simulink model "host_firmware_NVH_v6"  (R2022a)
settings: Solver=VariableStepAuto  StartTime=0.0  StopTime=Inf  RelTol=1e-3
InitFcn:
  | params_NVH;
undefined symbols (not defined in the file): denz, numz, Ts
libraries: simulink x8, instrumentseriallib x3
settings Model: Creator=Renato  LastModifiedBy=Renato
settings SolverCC: AlgebraicLoopSolver=TrustRegion
settings DebuggingCC: UnconnectedInputMsg=warning  UnconnectedOutputMsg=warning  UnconnectedLineMsg=warning  SFMachineParentedDataDiag=warning
settings RTWCC: DLArmComputeVersion=19.05

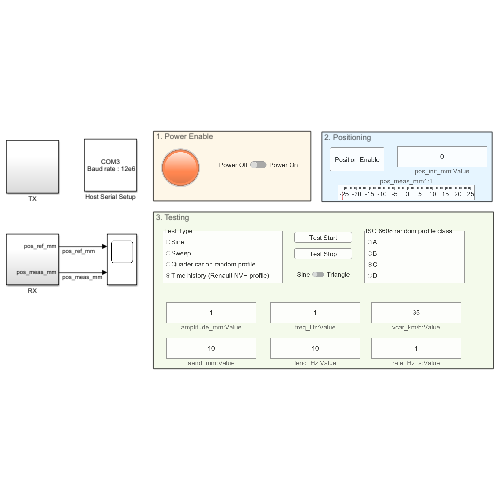
[thumbnail: Simulink's stored preview of the top-level diagram]
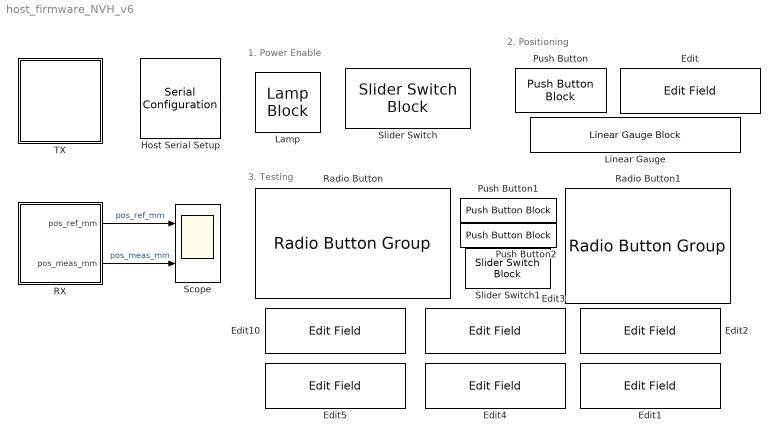
== system host_firmware_NVH_v6 ==
  note: 3. Testing
  note: 1. Power Enable
  note: 2. Positioning
  Edit{,1..5,10} (7 alike) : EditField  LabelPosition=Bottom  ShowInitialText=on  Alignment=Center
  Host Serial Setup : instrumentseriallib/Serial Configuration  Priority=-99  PortSel=COM3  Port=COM3  ComPort=COM3  BaudRate=12e6  DataBits=8  Parity=none  StopBits=1  ByteOrder=little-endian  FlowControl=none  Timeout=2  SimulateUsing=Interpreted execution  BlockInModel=on  aMode=5
      settings: SourceProductBaseCode=OT,IC,MT
  Lamp : LampBlock  LabelPosition=Hide
  Linear Gauge : LinearGaugeBlock  ScaleMin=-25  ScaleMax=25  TickInterval=5
  Push Button : PushButtonBlock  ButtonText=Position Enable  OffValue=0.000000
  Push Button1 : PushButtonBlock  ButtonText=Test Start  OffValue=0.000000
  Push Button2 : PushButtonBlock  ButtonText=Test Stop  OffValue=0.000000
  RX : Subsystem
  Radio Button : RadioButtonGroup  LabelPosition=Hide  SelectedLabel=Time history (Renault NVH profile)  ButtonGroupName=Test Type
      settings: Values={{'Sine', 'Sweep', 'Quarter car on random profile', 'Time history (Renault NVH profile)'}, [0 1 2 3]}
  Radio Button1 : RadioButtonGroup  LabelPosition=Hide  SelectedLabel=C  ButtonGroupName=ISO 8608 random profile class
      settings: Values={{'A', 'B', 'C', 'D'}, [0 1 2 3]}
  Scope : Scope  NumInputPorts=2
  Slider Switch : SliderSwitchBlock  LabelPosition=Hide
      settings: Values={{'Power Off', 'Power On'}, [0 1]}
  Slider Switch1 : SliderSwitchBlock  LabelPosition=Hide
      settings: Values={{'Sine', 'Triangle'}, [0 1]}
  TX : Subsystem
  wires:
  RX/1(pos_ref_mm) -> Scope/1  "pos_ref_mm"
  RX/2(pos_meas_mm) -> Scope/2  "pos_meas_mm"

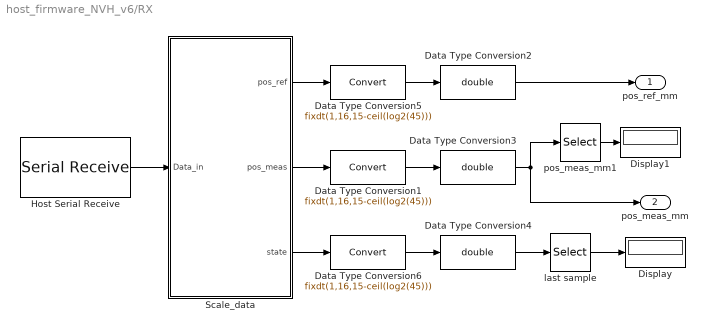
== system host_firmware_NVH_v6/RX ==
  Data Type Conversion1 : DataTypeConversion  OutDataTypeStr=fixdt(1,16,15-ceil(log2(45)))  ConvertRealWorld=Stored Integer (SI)  RndMeth=Simplest  SaturateOnIntegerOverflow=off
  Data Type Conversion2 : DataTypeConversion  OutDataTypeStr=double  RndMeth=Simplest  SaturateOnIntegerOverflow=off
  Data Type Conversion3 : DataTypeConversion  OutDataTypeStr=double  RndMeth=Simplest  SaturateOnIntegerOverflow=off
  Data Type Conversion4 : DataTypeConversion  OutDataTypeStr=double  RndMeth=Simplest  SaturateOnIntegerOverflow=off
  Data Type Conversion5 : DataTypeConversion  OutDataTypeStr=fixdt(1,16,15-ceil(log2(45)))  ConvertRealWorld=Stored Integer (SI)  RndMeth=Simplest  SaturateOnIntegerOverflow=off
  Data Type Conversion6 : DataTypeConversion  OutDataTypeStr=fixdt(1,16,15-ceil(log2(45)))  ConvertRealWorld=Stored Integer (SI)  RndMeth=Simplest  SaturateOnIntegerOverflow=off
  Display : Display
  Display1 : Display
  Host Serial Receive : instrumentseriallib/Serial Receive  PortSel=COM3  Port=COM3  ComPort=COM3  DataType=uint16  SaveDataType=uint8  ToggleHeader=on  Header='SS'  ToggleTerminator=on  Terminator=Custom terminator  CustomTerminator='EE'  InputFormat=Row major  ToggleDataSize=on  DataSize=[1000 3]  EnableBlockingMode=on  ActionDataUnavailable=Output last received value  ActionWhenDataUnavailable=Output last received value  CustomValue=0  SampleTime=1000 * Ts  SimulateUsing=Interpreted execution  BlockInModel=on  aMode=5
      settings: SourceProductBaseCode=OT,IC,MT
  Scale_data : MATLAB Function  TreatAsAtomicUnit=on
  last sample : Selector  NumberOfDimensions=2  InputPortWidth=3  IndexOptions=Index vector (dialog),Starting index (dialog)  Indices=1000,1  OutputSizes=1,1
  pos_meas_mm1 : Selector  NumberOfDimensions=2  InputPortWidth=3  IndexOptions=Index vector (dialog),Starting index (dialog)  Indices=1000,1  OutputSizes=1,1
  pos_ref_mm : Outport
  pos_meas_mm : Outport  Port=2
  wires:
  Host Serial Receive/1 -> Scale_data/1(Data_in)
  Scale_data/3(state) -> Data Type Conversion6/1
  Scale_data/2(pos_meas) -> Data Type Conversion1/1
  Scale_data/1(pos_ref) -> Data Type Conversion5/1
  Data Type Conversion5/1 -> Data Type Conversion2/1
  Data Type Conversion1/1 -> Data Type Conversion3/1
  Data Type Conversion2/1 -> pos_ref_mm/1
  Data Type Conversion3/1 -> pos_meas_mm1/1, pos_meas_mm/1
  Data Type Conversion4/1 -> last sample/1
  Data Type Conversion6/1 -> Data Type Conversion4/1
  last sample/1 -> Display/1
  pos_meas_mm1/1 -> Display1/1

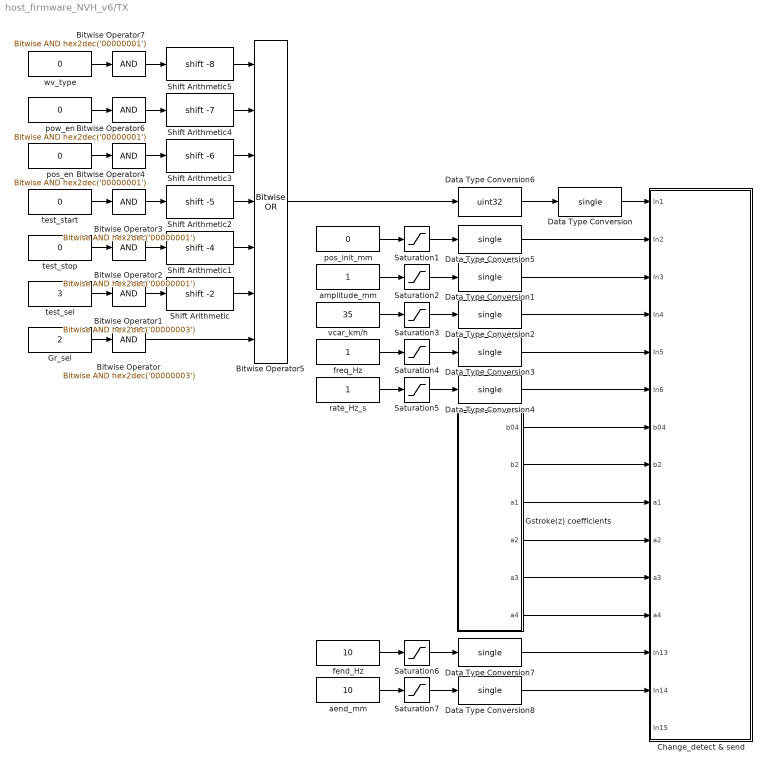
== system host_firmware_NVH_v6/TX ==
  Bitwise Operator : simulink/Logic and Bit Operations/Bitwise Operator  logicop=AND  UseBitMask=on  BitMask=hex2dec('00000003')  BitMaskRealWorld=Stored Integer
  Bitwise Operator1 : simulink/Logic and Bit Operations/Bitwise Operator  logicop=AND  UseBitMask=on  BitMask=hex2dec('00000003')  BitMaskRealWorld=Stored Integer
  Bitwise Operator{2..4,6..7} (5 alike) : simulink/Logic and Bit Operations/Bitwise Operator  logicop=AND  UseBitMask=on  BitMask=hex2dec('00000001')  BitMaskRealWorld=Stored Integer
  Bitwise Operator5 : simulink/Logic and Bit Operations/Bitwise Operator  logicop=OR  UseBitMask=off  NumInputPorts=7  BitMask=bin2dec('11011001')  BitMaskRealWorld=Stored Integer
  Change_detect & send : Subsystem
  Data Type Conversion : DataTypeConversion  OutDataTypeStr=single  ConvertRealWorld=Stored Integer (SI)  SaturateOnIntegerOverflow=off  RndMeth=Floor
  Data Type Conversion{1..5,7..8} (7 alike) : DataTypeConversion  OutDataTypeStr=single  RndMeth=Simplest  SaturateOnIntegerOverflow=off
  Data Type Conversion6 : DataTypeConversion  OutDataTypeStr=uint32  RndMeth=Simplest  SaturateOnIntegerOverflow=off
  Gr_sel : Constant  Value=2  VectorParams1D=off  OutDataTypeStr=uint32  SampleTime=0.01
  Gstroke(z) coefficients : Subsystem
  Saturation1 : Saturate  UpperLimit=20  LowerLimit=-20
  Saturation2 : Saturate  UpperLimit=20  LowerLimit=0
  Saturation3 : Saturate  UpperLimit=200  LowerLimit=10
  Saturation4 : Saturate  UpperLimit=100  LowerLimit=0.1
  Saturation5 : Saturate  UpperLimit=10  LowerLimit=0.1
  Saturation6 : Saturate  UpperLimit=100  LowerLimit=0.1
  Saturation7 : Saturate  UpperLimit=20  LowerLimit=0
  Shift Arithmetic : ArithShift  BitShiftNumber=-2
  Shift Arithmetic1 : ArithShift  BitShiftNumber=-4
  Shift Arithmetic2 : ArithShift  BitShiftNumber=-5
  Shift Arithmetic3 : ArithShift  BitShiftNumber=-6
  Shift Arithmetic4 : ArithShift  BitShiftNumber=-7
  Shift Arithmetic5 : ArithShift  BitShiftNumber=-8
  aend_mm : Constant  Value=10  VectorParams1D=off  OutDataTypeStr=single  SampleTime=0.01
  amplitude_mm : Constant  VectorParams1D=off  OutDataTypeStr=single  SampleTime=0.01
  fend_Hz : Constant  Value=10  VectorParams1D=off  OutDataTypeStr=single  SampleTime=0.01
  freq_Hz : Constant  VectorParams1D=off  OutDataTypeStr=single  SampleTime=0.01
  pos_en : Constant  Value=0  VectorParams1D=off  OutDataTypeStr=uint32  SampleTime=0.01
  pos_init_mm : Constant  Value=0  VectorParams1D=off  OutDataTypeStr=single  SampleTime=0.01
  pow_en : Constant  Value=0  VectorParams1D=off  OutDataTypeStr=uint32  SampleTime=0.01
  rate_Hz_s : Constant  VectorParams1D=off  OutDataTypeStr=single  SampleTime=0.01
  test_sel : Constant  Value=3  VectorParams1D=off  OutDataTypeStr=uint32  SampleTime=0.01
  test_start : Constant  Value=0  VectorParams1D=off  OutDataTypeStr=uint32  SampleTime=0.01
  test_stop : Constant  Value=0  VectorParams1D=off  OutDataTypeStr=uint32  SampleTime=0.01
  vcar_km/h : Constant  Value=35  VectorParams1D=off  OutDataTypeStr=single  SampleTime=0.01
  wv_type : Constant  Value=0  VectorParams1D=off  OutDataTypeStr=uint32  SampleTime=0.01
  wires:
  test_sel/1 -> Bitwise Operator1/1
  Gr_sel/1 -> Bitwise Operator/1
  Bitwise Operator1/1 -> Shift Arithmetic/1
  test_stop/1 -> Bitwise Operator2/1
  test_start/1 -> Bitwise Operator3/1
  pos_en/1 -> Bitwise Operator4/1
  pow_en/1 -> Bitwise Operator6/1
  Bitwise Operator2/1 -> Shift Arithmetic1/1
  Bitwise Operator3/1 -> Shift Arithmetic2/1
  Bitwise Operator4/1 -> Shift Arithmetic3/1
  Bitwise Operator6/1 -> Shift Arithmetic4/1
  pos_init_mm/1 -> Saturation1/1
  amplitude_mm/1 -> Saturation2/1
  vcar_km/h/1 -> Saturation3/1
  freq_Hz/1 -> Saturation4/1
  Saturation2/1 -> Data Type Conversion1/1
  Saturation3/1 -> Data Type Conversion2/1
  Saturation4/1 -> Data Type Conversion3/1
  Saturation1/1 -> Data Type Conversion5/1
  Bitwise Operator5/1 -> Data Type Conversion6/1
  Data Type Conversion/1 -> Change_detect & send/1(In1)
  Saturation5/1 -> Data Type Conversion4/1
  rate_Hz_s/1 -> Saturation5/1
  Data Type Conversion5/1 -> Change_detect & send/2(In2)
  Data Type Conversion1/1 -> Change_detect & send/3(In3)
  Data Type Conversion2/1 -> Change_detect & send/4(In4)
  Data Type Conversion3/1 -> Change_detect & send/5(In5)
  Data Type Conversion4/1 -> Change_detect & send/6(In6)
  Gstroke(z) coefficients/1(b04) -> Change_detect & send/7(b04)
  Gstroke(z) coefficients/2(b2) -> Change_detect & send/8(b2)
  Gstroke(z) coefficients/3(a1) -> Change_detect & send/9(a1)
  Gstroke(z) coefficients/4(a2) -> Change_detect & send/10(a2)
  Gstroke(z) coefficients/5(a3) -> Change_detect & send/11(a3)
  Gstroke(z) coefficients/6(a4) -> Change_detect & send/12(a4)
  Data Type Conversion6/1 -> Data Type Conversion/1
  Data Type Conversion7/1 -> Change_detect & send/13(In13)
  Saturation6/1 -> Data Type Conversion7/1
  fend_Hz/1 -> Saturation6/1
  Data Type Conversion8/1 -> Change_detect & send/14(In14)
  aend_mm/1 -> Saturation7/1
  Saturation7/1 -> Data Type Conversion8/1
  Bitwise Operator/1 -> Bitwise Operator5/7
  wv_type/1 -> Bitwise Operator7/1
  Bitwise Operator7/1 -> Shift Arithmetic5/1
  Shift Arithmetic5/1 -> Bitwise Operator5/1
  Shift Arithmetic4/1 -> Bitwise Operator5/2
  Shift Arithmetic3/1 -> Bitwise Operator5/3
  Shift Arithmetic2/1 -> Bitwise Operator5/4
  Shift Arithmetic1/1 -> Bitwise Operator5/5
  Shift Arithmetic/1 -> Bitwise Operator5/6

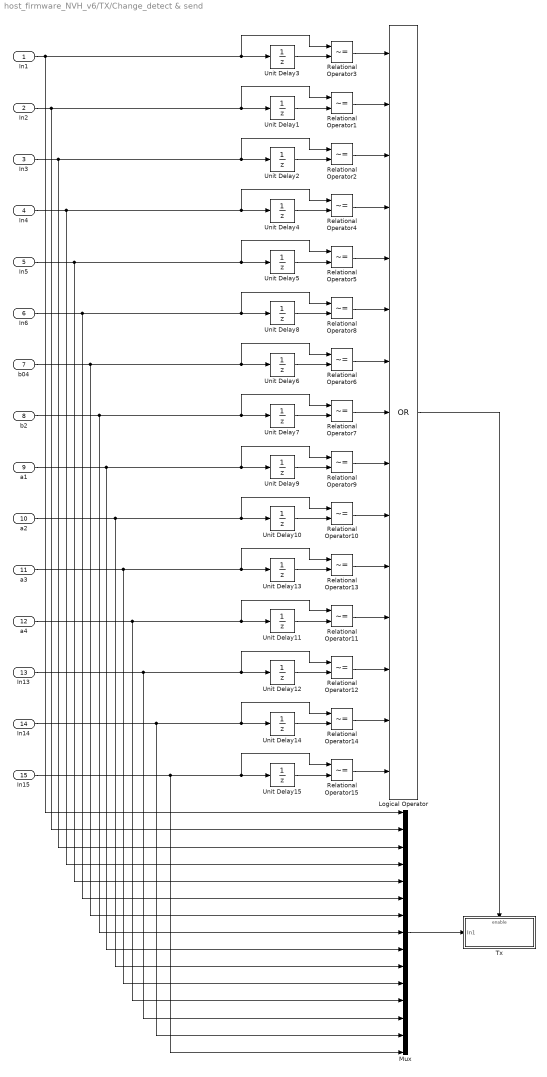
== system host_firmware_NVH_v6/TX/Change_detect & send ==
  In1 : Inport
  In2 : Inport  Port=2
  In3 : Inport  Port=3
  In4 : Inport  Port=4
  In5 : Inport  Port=5
  In6 : Inport  Port=6
  b04 : Inport  Port=7
  b2 : Inport  Port=8
  a1 : Inport  Port=9
  a2 : Inport  Port=10
  a3 : Inport  Port=11
  a4 : Inport  Port=12
  In13 : Inport  Port=13
  In14 : Inport  Port=14
  In15 : Inport  Port=15
  Logical Operator : Logic  Operator=OR  Inputs=15  AllPortsSameDT=off  OutDataTypeStr=boolean
  Mux : Mux  Inputs=15
  Relational Operator{1..15} (15 alike) : RelationalOperator  Operator=~=  OutDataTypeStr=boolean  InputSameDT=off
  Tx : Subsystem  TreatAsAtomicUnit=on
  Unit Delay{1..15} (15 alike) : UnitDelay  SampleTime=-1  HasFrameUpgradeWarning=on
  wires:
  In2/1 -> Relational Operator1/1, Unit Delay1/1, Mux/2
  Relational Operator1/1 -> Logical Operator/2
  Unit Delay1/1 -> Relational Operator1/2
  Relational Operator3/1 -> Logical Operator/1
  Unit Delay2/1 -> Relational Operator2/2
  Relational Operator2/1 -> Logical Operator/3
  In3/1 -> Relational Operator2/1, Unit Delay2/1, Mux/3
  Unit Delay3/1 -> Relational Operator3/2
  In1/1 -> Relational Operator3/1, Unit Delay3/1, Mux/1
  In4/1 -> Relational Operator4/1, Unit Delay4/1, Mux/4
  Unit Delay4/1 -> Relational Operator4/2
  Relational Operator4/1 -> Logical Operator/4
  In5/1 -> Relational Operator5/1, Unit Delay5/1, Mux/5
  Unit Delay5/1 -> Relational Operator5/2
  Relational Operator5/1 -> Logical Operator/5
  Relational Operator8/1 -> Logical Operator/6
  Relational Operator10/1 -> Logical Operator/10
  Unit Delay9/1 -> Relational Operator9/2
  Unit Delay10/1 -> Relational Operator10/2
  In6/1 -> Relational Operator8/1, Unit Delay8/1, Mux/6
  Unit Delay7/1 -> Relational Operator7/2
  a1/1 -> Mux/9, Relational Operator9/1, Unit Delay9/1
  Unit Delay6/1 -> Relational Operator6/2
  a2/1 -> Mux/10, Relational Operator10/1, Unit Delay10/1
  b2/1 -> Mux/8, Relational Operator7/1, Unit Delay7/1
  Unit Delay8/1 -> Relational Operator8/2
  Relational Operator9/1 -> Logical Operator/9
  b04/1 -> Mux/7, Relational Operator6/1, Unit Delay6/1
  Relational Operator7/1 -> Logical Operator/8
  Relational Operator6/1 -> Logical Operator/7
  Relational Operator13/1 -> Logical Operator/11
  Relational Operator15/1 -> Logical Operator/15
  Unit Delay14/1 -> Relational Operator14/2
  Unit Delay15/1 -> Relational Operator15/2
  a3/1 -> Mux/11, Relational Operator13/1, Unit Delay13/1
  Unit Delay12/1 -> Relational Operator12/2
  In14/1 -> Mux/14, Relational Operator14/1, Unit Delay14/1
  Unit Delay11/1 -> Relational Operator11/2
  In15/1 -> Mux/15, Relational Operator15/1, Unit Delay15/1
  In13/1 -> Mux/13, Relational Operator12/1, Unit Delay12/1
  Unit Delay13/1 -> Relational Operator13/2
  Relational Operator14/1 -> Logical Operator/14
  a4/1 -> Mux/12, Relational Operator11/1, Unit Delay11/1
  Relational Operator12/1 -> Logical Operator/13
  Relational Operator11/1 -> Logical Operator/12
  Logical Operator/1 -> Tx/Enable
  Mux/1 -> Tx/1(In1)

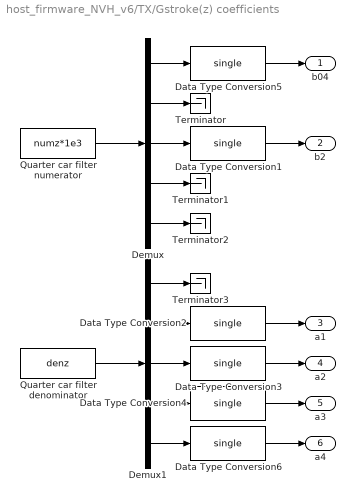
== system host_firmware_NVH_v6/TX/Gstroke(z) coefficients ==
  Data Type Conversion{1..6} (6 alike) : DataTypeConversion  OutDataTypeStr=single  RndMeth=Simplest  SaturateOnIntegerOverflow=off
  Demux : Demux  Outputs=5
  Demux1 : Demux  Outputs=5
  Quarter car filter denominator : Constant  Value=denz  VectorParams1D=off  OutDataTypeStr=double  SampleTime=0.01
  Quarter car filter numerator : Constant  Value=numz*1e3  VectorParams1D=off  OutDataTypeStr=double  SampleTime=0.01
  Terminator{,1..3} (4 alike) : Terminator
  b04 : Outport
  b2 : Outport  Port=2
  a1 : Outport  Port=3
  a2 : Outport  Port=4
  a3 : Outport  Port=5
  a4 : Outport  Port=6
  wires:
  Demux/4 -> Terminator1/1
  Quarter car filter denominator/1 -> Demux1/1
  Demux/3 -> Data Type Conversion1/1
  Quarter car filter numerator/1 -> Demux/1
  Demux1/3 -> Data Type Conversion3/1
  Demux/1 -> Data Type Conversion5/1
  Demux1/2 -> Data Type Conversion2/1
  Demux1/4 -> Data Type Conversion4/1
  Data Type Conversion4/1 -> a3/1
  Demux/2 -> Terminator/1
  Demux/5 -> Terminator2/1
  Data Type Conversion6/1 -> a4/1
  Demux1/5 -> Data Type Conversion6/1
  Demux1/1 -> Terminator3/1
  Data Type Conversion3/1 -> a2/1
  Data Type Conversion1/1 -> b2/1
  Data Type Conversion5/1 -> b04/1
  Data Type Conversion2/1 -> a1/1

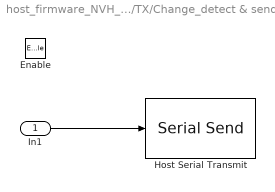
== system host_firmware_NVH_v6/TX/Change_detect & send/Tx ==
  In1 : Inport
  Enable : EnablePort
  Host Serial Transmit : instrumentseriallib/Serial Send  PortSel=COM3  Port=COM3  ComPort=COM3  Header=[]  Terminator=<none>  CustomTerminator=[]  EnableBlockingMode=off  SimulateUsing=Interpreted execution  BlockInModel=on  aMode=5
      settings: SourceProductBaseCode=OT,IC,MT
  wires:
  In1/1 -> Host Serial Transmit/1

== matlab function host_firmware_NVH_v6/RX/Scale_data ==
  data: pos_ref output; pos_meas output; state output; Data_in input
function [pos_ref,pos_meas,state]  = unBuf(Data_in)
pos_ref = Data_in(:, 1);
pos_meas = Data_in(:, 2);
state = Data_in(:, 3);
end
